simulink model "Model_of_crane"  (R2022b)
settings: Solver=VariableStepAuto  StartTime=0.0  StopTime=10.0  FixedStep=0.01  RelTol=1e-3
undefined symbols (not defined in the file or in its folder): b_rot, bp, g, Jm, Jp, Ke, Kt, Lcm, Lr, ml, mr, ms, Ra, rm
settings Model: Creator=TJ  LastModifiedBy=TJ

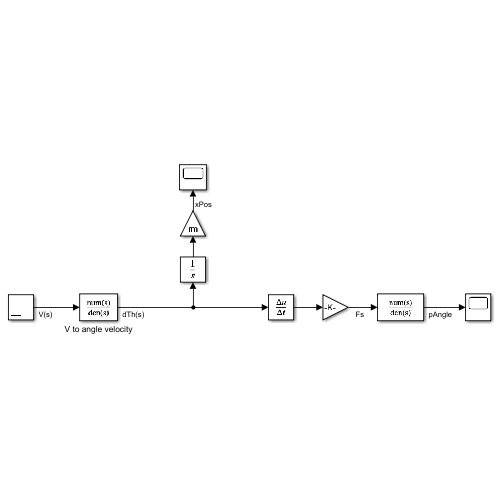
[thumbnail: Simulink's stored preview of the top-level diagram]
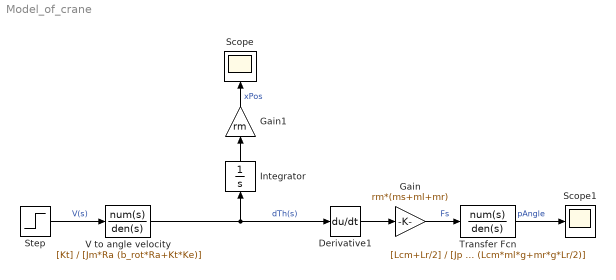
== system Model_of_crane ==
  Derivative1 : Derivative
  Gain : Gain  Gain=rm*(ms+ml+mr)
  Gain1 : Gain  Gain=rm
  Integrator : Integrator
  Scope : Scope
  Scope1 : Scope
  Step : Step  SampleTime=0
  Transfer Fcn : TransferFcn  Numerator=[Lcm+Lr/2]  Denominator=[Jp bp (Lcm*ml*g+mr*g*Lr/2)]
  V to angle velocity : TransferFcn  Numerator=[Kt]  Denominator=[Jm*Ra (b_rot*Ra+Kt*Ke)]
  wires:
  Gain1/1 -> Scope/1  "xPos"
  Gain/1 -> Transfer Fcn/1  "Fs"
  Step/1 -> V to angle velocity/1  "V(s)"
  V to angle velocity/1 -> Derivative1/1, Integrator/1  "dTh(s)"
  Derivative1/1 -> Gain/1
  Integrator/1 -> Gain1/1
  Transfer Fcn/1 -> Scope1/1  "pAngle"
